simulink model "Control_DC_DC_Test"  (R2018b)
settings: Solver=FixedStepDiscrete  StartTime=0.0  StopTime=1  RelTol=1e-3
undefined symbols (not defined in the file): sigbuilder_block
libraries: powerlib x32, re_lib x1, powerlib_meascontrol x1
settings Model: Creator=jasil  LastModifiedBy=mwkane

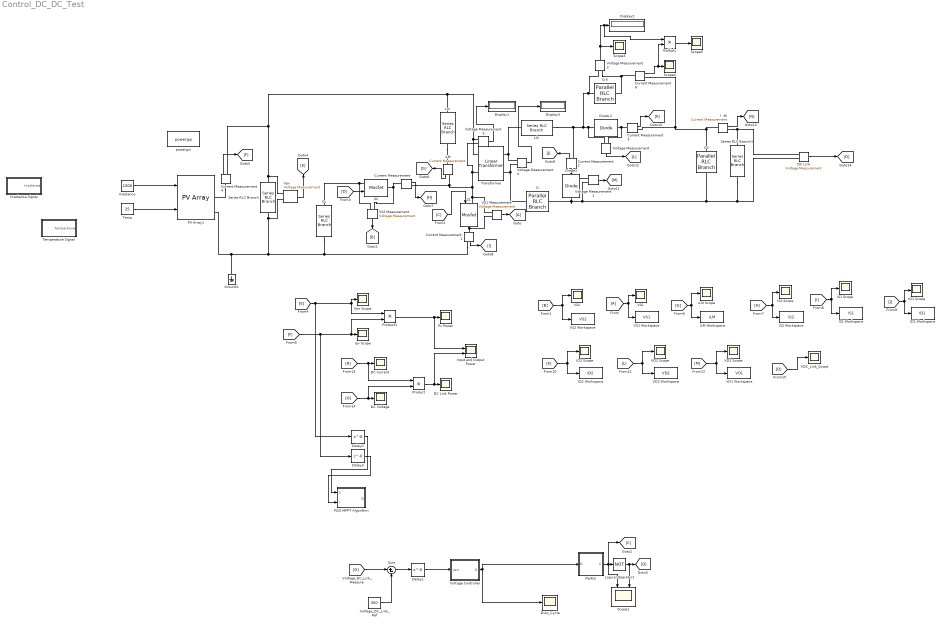
== system Control_DC_DC_Test ==
  " Cd" : powerlib/Elements/Parallel RLC Branch  LConnTagsString=a  RConnTagsString=__new0  BranchType=C  Resistance=1  Inductance=1e-3  SetiL0=off  InitialCurrent=0  Capacitance=1e-5  Setx0=off  InitialVoltage=0  Measurements=None
      settings: SourceProductName=Simscape Electrical
  Cc : powerlib/Elements/Series RLC Branch  LConnTagsString=__new0  RConnTagsString=__new0  BranchType=RC  Resistance=0.001  Inductance=1e-3  SetiL0=off  InitialCurrent=0  Capacitance=2.2e-6  Setx0=off  InitialVoltage=0  Measurements=None
      settings: SourceProductName=Simscape Electrical
  Cr : powerlib/Elements/Parallel RLC Branch  LConnTagsString=a  RConnTagsString=__new0  BranchType=C  Resistance=1  Inductance=1e-3  SetiL0=off  InitialCurrent=0  Capacitance=2.4e-6  Setx0=off  InitialVoltage=0  Measurements=None
      settings: SourceProductName=Simscape Electrical
  Cr3 : powerlib/Elements/Parallel RLC Branch  LConnTagsString=a  RConnTagsString=__new0  BranchType=R  Resistance=1e3  Inductance=2.6e-6  SetiL0=off  InitialCurrent=0  Capacitance=2.4e-6  Setx0=off  InitialVoltage=0  Measurements=None
      settings: SourceProductName=Simscape Electrical
  Current Measurement{,1..4,6} (6 alike) : powerlib/Measurements/Current Measurement  PhasorSimulation=off  OutputType=Complex  PSBequivalent=0
      settings: SourceProductName=Simscape Electrical
  DC Current : Scope
  DC Link : powerlib/Measurements/Voltage Measurement  PhasorSimulation=off  OutputType=Complex  PSBequivalent=0
      settings: SourceProductName=Simscape Electrical
  DC Link Power : Scope
  DC Voltage : Scope
  Delay1 : Delay  DelayLength=0  SampleTime=0.0001
  Delay2 : Delay  DelayLength=0  SampleTime=0.001
  Delay3 : Delay  DelayLength=0  SampleTime=0.001
  Diode 2 : powerlib/Power Electronics/Diode  Ron=1  Lon=0  Vf=0.8  IC=0  UseSnubber=0  Rs=inf  Cs=0  Measurements=off
      settings: SourceProductName=Simscape Electrical
  Diode1 : powerlib/Power Electronics/Diode  Ron=0.01  Lon=0  Vf=0.8  IC=0  UseSnubber=0  Rs=inf  Cs=0  Measurements=off
      settings: SourceProductName=Simscape Electrical
  Display1 : Display
  Display2 : Display
  Display3 : Display
  Duty_Cycle : Scope
  Ground1 : powerlib/Elements/Ground  LConnTagsString=a
      settings: SourceProductName=Simscape Electrical
  I  dc : powerlib/Measurements/Current Measurement  PhasorSimulation=off  OutputType=Complex  PSBequivalent=0
      settings: SourceProductName=Simscape Electrical
  ID1 Scope : Scope
  ID1 Workspace : ToWorkspace  VariableName=ID1  SaveFormat=Timeseries  SampleTime=-1
  ID2 Scope : Scope
  ID2 Workspace : ToWorkspace  VariableName=ID2  SaveFormat=Timeseries  SampleTime=-1
  ILM Workspace : ToWorkspace  VariableName=ILM  SaveFormat=Timeseries  SampleTime=-1
  IS1 Scope : Scope
  IS1 Workspace : ToWorkspace  VariableName=IS1  SaveFormat=Timeseries  SampleTime=-1
  IS2 Scope : Scope
  IS2 Workspace : ToWorkspace  VariableName=IS2  SaveFormat=Timeseries  SampleTime=-1
  Input and Output Power : Scope  NumInputPorts=2
  Ipv Scope : Scope
  Irradiance : Constant  Value=1000
  "Irradiance Signal " : Subsystem  Tag=STV Subsys  LoadFcn=sigbuilder_block('load');  StartFcn=sigbuilder_block('start');  StopFcn=sigbuilder_block('stop');  ClipboardFcn=sigbuilder_block('clipboard');  mask(Sigbuilder block){tuvar=[0:10]}
      mask help: Simulink:masks:SigbuilderBlock_MD
      mask init:
      | if ~strcmp(get_param(bdroot(gcbh),'SimulationStatus'),'stopped') tuvar = sigbuilder_block('maskInit'); end
      settings: CopyFcn=sigbuilder_block('copy');  DeleteFcn=sigbuilder_block('delete');  ModelCloseFcn=sigbuilder_block('modelClose');  PreSaveFcn=sigbuilder_block('preSave');  PauseFcn=sigbuilder_block('pause');  ContinueFcn=sigbuilder_block('continue');  NameChangeFcn=sigbuilder_block('namechange');  OpenFcn=sigbuilder_block('open',[6 30 1012.5 447.75 ]);  CloseFcn=sigbuilder_block('close');
      mask Display: plot(0, 0, 100, 100,[2, 2, 32, 32, 2], [68, 8, 8, 68, 68],[32, 2], [38, 38], [32, 19, 2],[53, 60, 44], [32, 17, 17, 2],[16, 16, 31, 31]);txt = getActiveGroup(gcbh);text(2, 100, txt,'verticalAlignment', 'top');
  Llk : powerlib/Elements/Series RLC Branch  LConnTagsString=__new0  RConnTagsString=__new0  BranchType=RL  Resistance=0.001  Inductance=2.6e-6  SetiL0=off  InitialCurrent=0  Capacitance=1e-6  Setx0=off  InitialVoltage=0  Measurements=None
      settings: SourceProductName=Simscape Electrical
  Lm : powerlib/Elements/Series RLC Branch  LConnTagsString=__new0  RConnTagsString=__new0  BranchType=RL  Resistance=0.001  Inductance=20e-6  SetiL0=off  InitialCurrent=0  Capacitance=1e-6  Setx0=off  InitialVoltage=0  Measurements=None
      settings: SourceProductName=Simscape Electrical
  Logical Operator1 : Logic  Operator=NOT  AllPortsSameDT=off  OutDataTypeStr=boolean
  Multiply : Product
  P&O MPPT Algorithm : MATLAB Function  TreatAsAtomicUnit=on
  PV Array1 : re_lib/Solar/PV Array  Npar=1  Nser=2  PlotType=array @ 25 deg.C & specified irradiances  S_vec="[ 1000  500  100 ]"  Temp_C_vec="[ 45 25  ]"  ModuleName=User-defined  PlotWhenSelected=off  Pm=179.9805  Ncell=36  Voc=24.06  Isc=9.77  Vm=19.67  Im=9.15  beta_Voc_pc=-0.28  alpha_Isc_pc=+0.04  beta_Voc=-0.067368  alpha_Isc=0.003908  IL=9.8911  I0=1.3829e-11  nI=0.95443  Rsh=60.4787  Rs=0.18212  BAL=off  Tc=1e-6  Tfilter=5e-5
      settings: SourceProductName=Simscape Electrical
  PWM2 : Subsystem
  Product : Product
  Product1 : Product
  Pv Power : Scope
  S1 : powerlib/Power Electronics/Mosfet  Ron=5.6e-3  Lon=0  Rd=0.01  Vfd=1.3  IC=0  Rs=1e6  Cs=inf  Measurements=off
      settings: SourceProductName=Simscape Electrical
  S2 : powerlib/Power Electronics/Mosfet  Ron=5.6e-3  Lon=0  Rd=0.01  Vfd=1.3  IC=0  Rs=1e5  Cs=inf  Measurements=off
      settings: SourceProductName=Simscape Electrical
  Scope1 : Scope  NumInputPorts=2
  Scope3 : Scope
  Scope4 : Scope
  Scope5 : Scope
  Series RLC Branch : powerlib/Elements/Series RLC Branch  LConnTagsString=__new0  RConnTagsString=__new0  BranchType=RC  Resistance=0.000001  Inductance=1e-3  SetiL0=off  InitialCurrent=0  Capacitance=1e-3  Setx0=off  InitialVoltage=0  Measurements=Branch voltage
      settings: SourceProductName=Simscape Electrical
  Series RLC Branch1 : powerlib/Elements/Series RLC Branch  LConnTagsString=__new0  RConnTagsString=__new0  BranchType=R  Resistance=695  Inductance=1e-3  SetiL0=off  InitialCurrent=0  Capacitance=1e-6  Setx0=off  InitialVoltage=0  Measurements=None
      settings: SourceProductName=Simscape Electrical
  Sum : Sum  Inputs=|+-
  Temp : Constant  Value=25
  Temperature Signal : Subsystem  Tag=STV Subsys  LoadFcn=sigbuilder_block('load');  StartFcn=sigbuilder_block('start');  StopFcn=sigbuilder_block('stop');  ClipboardFcn=sigbuilder_block('clipboard');  mask(Sigbuilder block){tuvar=[0:10]}
      mask help: Simulink:masks:SigbuilderBlock_MD
      mask init:
      | if ~strcmp(get_param(bdroot(gcbh),'SimulationStatus'),'stopped') tuvar = sigbuilder_block('maskInit'); end
      settings: CopyFcn=sigbuilder_block('copy');  DeleteFcn=sigbuilder_block('delete');  ModelCloseFcn=sigbuilder_block('modelClose');  PreSaveFcn=sigbuilder_block('preSave');  PauseFcn=sigbuilder_block('pause');  ContinueFcn=sigbuilder_block('continue');  NameChangeFcn=sigbuilder_block('namechange');  OpenFcn=sigbuilder_block('open',[6 30 1012.5 447.75 ]);  CloseFcn=sigbuilder_block('close');
      mask Display: plot(0, 0, 100, 100,[2, 2, 32, 32, 2], [68, 8, 8, 68, 68],[32, 2], [38, 38], [32, 19, 2],[53, 60, 44], [32, 17, 17, 2],[16, 16, 31, 31]);txt = getActiveGroup(gcbh);text(2, 100, txt,'verticalAlignment', 'top');
  Transformer : powerlib/Elements/Linear Transformer  UNITS=SI  NominalPower=[ 25 100e3 ]  winding1=[9 0 0]  winding2=[38 0 0]  ThreeWindings=off  winding3=[3.15e+05 3.969e+07 6316.9]  RmLm=[1e6 0]  Measurements=Magnetization current  DataType=on
      settings: SourceProductName=Simscape Electrical
  VD1 Scope : Scope
  VD1 Workspace : ToWorkspace  VariableName=VD1  SaveFormat=Timeseries  SampleTime=-1
  VD2 Scope : Scope
  VD2 Workspace : ToWorkspace  VariableName=VD2  SaveFormat=Timeseries  SampleTime=-1
  VDC_Link_Scope : Scope
  VS1 : Scope
  VS1 Measurement : powerlib/Measurements/Voltage Measurement  PhasorSimulation=off  OutputType=Complex  PSBequivalent=0
      settings: SourceProductName=Simscape Electrical
  VS1 Workspace : ToWorkspace  VariableName=VS1  SaveFormat=Timeseries  SampleTime=-1
  VS2 : Scope
  VS2 Measurement : powerlib/Measurements/Voltage Measurement  PhasorSimulation=off  OutputType=Complex  PSBequivalent=0
      settings: SourceProductName=Simscape Electrical
  VS2 Workspace : ToWorkspace  VariableName=VS2  SaveFormat=Timeseries  SampleTime=-1
  Voltage Controller : MATLAB Function  TreatAsAtomicUnit=on
  Voltage Measurement{,1..4} (5 alike) : powerlib/Measurements/Voltage Measurement  PhasorSimulation=off  OutputType=Complex  PSBequivalent=0
      settings: SourceProductName=Simscape Electrical
  Voltage_DC_Link_Ref : Constant  Value=350
  Vpv : powerlib/Measurements/Voltage Measurement  PhasorSimulation=off  OutputType=Complex  PSBequivalent=0
      settings: SourceProductName=Simscape Electrical
  Vpv Scope : Scope
  iLM : powerlib/Measurements/Current Measurement  PhasorSimulation=off  OutputType=Complex  PSBequivalent=0
      settings: SourceProductName=Simscape Electrical
  iLM Scope : Scope
  powergui : powerlib/powergui  Priority=1  SimulationMode=Discrete  SampleTime=50e-9  frequency=60  Iterations=50  frequencyindice=0  Pbase=100e6  ErrMax=1e-4  UnitsV=kV  UnitsW=MW  buscounter=0  FunctionMessages=off  echomessages=off  EnableUseOfTLC=off  CurrentSourceSwitches=off  DisableSnubberDevices=off  DisableRonSwitches=off  DisableVfSwitches=off  DisplayEquations=off  SolverType=Tustin/Backward Euler (TBE)  Interpol=off  ExternalGateDelay=off  methode=off  Ts=100  x0status=blocks  SPID=on  SwTol=0  HookPort=off  RestoreLinks=warning  ResistiveCurrentMeasurement=off  Frange=[0:2:500]  Ylog=off  Xlog=on  ShowGrid=off  save=off  variable=ZData  structure=0  ZoomFFT=off  StartTime=0.0  cycles=1  DisplayStyle=1  fundamental=60  FreqAxis=off  MaxFrequency=1000  frequencyindicesteady=1  RmsSteady=1  display=off
      settings: SourceProductName=Simscape Electrical
  wires:
  Product1/1 -> Input and Output Power/1, Pv Power/1
  Delay2/1 -> P&O MPPT Algorithm/1(V)
  Delay3/1 -> P&O MPPT Algorithm/2(I)
  PWM2/1(S) -> Scope1/1, [C], Logical Operator1/1
  VS1 Measurement/1 -> [A]
  [A] -> VS1 Workspace/1, VS1/1
  VS2 Measurement/1 -> [B]
  [B] -> VS2 Workspace/1, VS2/1
  Logical Operator1/1 -> Scope1/2, [D]
  [C] -> S1/1
  [D] -> S2/1
  [E] -> Delay2/1, Vpv Scope/1, Product1/1
  [F] -> Product1/2, Ipv Scope/1, Delay3/1
  iLM/1 -> [G]
  [G] -> iLM Scope/1, ILM Workspace/1
  Current Measurement/1 -> [H]
  [H] -> IS2 Workspace/1, IS2 Scope/1
  Current Measurement1/1 -> [I]
  [I] -> IS1 Workspace/1, IS1 Scope/1
  Current Measurement2/1 -> [J]
  [J] -> ID1 Workspace/1, ID1 Scope/1
  Current Measurement3/1 -> [K]
  [K] -> ID2 Workspace/1, ID2 Scope/1
  [L] -> VD2 Workspace/1, VD2 Scope/1
  [M] -> VD1 Workspace/1, VD1 Scope/1
  Voltage Measurement/1 -> [L]
  Voltage Measurement1/1 -> [M]
  DC Link/1 -> [O]
  Vpv/1 -> [E]
  Current Measurement4/1 -> [F]
  I  dc/1 -> [N]
  Product/1 -> Input and Output Power/2, DC Link Power/1
  [O] -> Product/2, DC Voltage/1
  [N] -> Product/1, DC Current/1
  Voltage Measurement2/1 -> Scope3/1, Multiply/1, Display2/1
  Current Measurement6/1 -> Multiply/2, Scope4/1
  Multiply/1 -> Scope5/1
  Voltage Measurement3/1 -> Display1/1
  Voltage Measurement4/1 -> Display3/1
  [O] -> Sum/1
  Voltage_DC_Link_Ref/1 -> Sum/2
  Sum/1 -> Delay1/1
  Delay1/1 -> Voltage Controller/1(Verr)
  Voltage Controller/1(D) -> PWM2/1(D), Duty_Cycle/1
  [O] -> VDC_Link_Scope/1
  Irradiance/1 -> PV Array1/1
  Temp/1 -> PV Array1/2
  connections:
  Current Measurement3/RConn1 -- Current Measurement6/RConn1 -- I  dc/LConn1 -- " Cd"/LConn1
  S1/LConn1 -- VS1 Measurement/LConn1 -- Voltage Measurement3/LConn2 -- Transformer/LConn2 -- Current Measurement/RConn1 -- iLM/RConn1
  Cr/RConn1 -- Voltage Measurement1/LConn2 -- " Cd"/RConn1 -- DC Link/LConn2 -- Series RLC Branch1/RConn1 -- Diode1/LConn1
  Transformer/LConn1 -- Voltage Measurement3/LConn1 -- Lm/LConn1 -- Current Measurement4/RConn1 -- Vpv/LConn1 -- Series RLC Branch/LConn1
  Current Measurement1/RConn1 -- Cc/RConn1 -- Vpv/LConn2 -- Series RLC Branch/RConn1 -- Ground1/LConn1 -- PV Array1/RConn2
  Cr3/LConn1 -- Voltage Measurement2/LConn1 -- Llk/RConn1 -- Current Measurement2/RConn1 -- Voltage Measurement/LConn2 -- Diode 2/LConn1
  I  dc/RConn1 -- Series RLC Branch1/LConn1 -- DC Link/LConn1
  VS2 Measurement/LConn1 -- Cc/LConn1 -- S2/LConn1
  Cr/LConn1 -- Voltage Measurement4/LConn2 -- Transformer/RConn2
  Lm/RConn1 -- iLM/LConn1
  VS2 Measurement/LConn2 -- Current Measurement/LConn1 -- S2/RConn1
  Current Measurement1/LConn1 -- S1/RConn1 -- VS1 Measurement/LConn2
  Current Measurement2/LConn1 -- Diode1/RConn1 -- Voltage Measurement1/LConn1
  Current Measurement3/LConn1 -- Voltage Measurement/LConn1 -- Diode 2/RConn1
  Current Measurement4/LConn1 -- PV Array1/RConn1
  Llk/LConn1 -- Voltage Measurement4/LConn1 -- Transformer/RConn1
  Voltage Measurement2/LConn2 -- Cr3/RConn1 -- Current Measurement6/LConn1

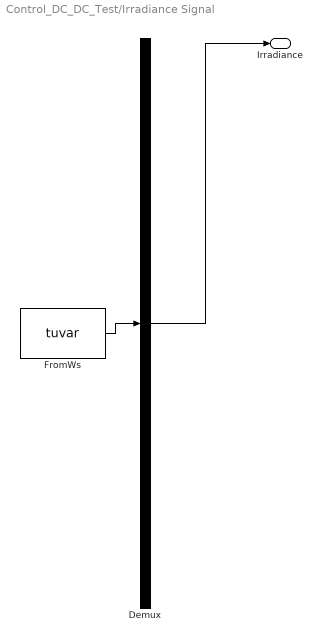
== system Control_DC_DC_Test/Irradiance Signal  ==
  Demux : Demux  Tag=STV Demux  Outputs=1
  FromWs : FromWorkspace  Tag=STV FromWs  VariableName=tuvar  SampleTime=0
      SigBuilderData=|
      | common.afterFinalStr = 'Extrapolate'
      | common.sampleTime = 0
      | dataSet.timeRange = [0 0.3]
      | dataSet.name = 'Group 1'
      | sbobj.Groups.Name = 'Group 1'
      | sbobj.Groups.Signals.Name = 'Irradiance'
      | sbobj.Groups.Signals.XData = [0 0.1 0.1 0.2 0.2 0.3]
      | sbobj.Groups.Signals.YData = [1000 1000 500 500 1000 1000]
      | sbobj.Groups.TimeRange = [0 0.3]
  Irradiance : Outport  Tag=STV Outport
  wires:
  Demux/1 -> Irradiance/1
  FromWs/1 -> Demux/1

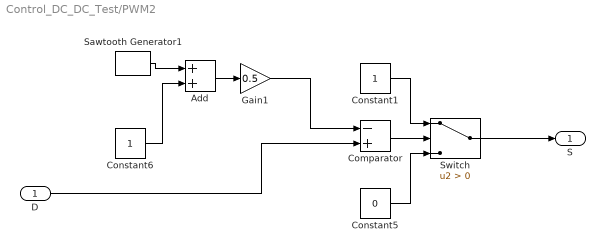
== system Control_DC_DC_Test/PWM2 ==
  D : Inport
  Add : Sum
  Comparator : Sum  Inputs=-+
  Constant1 : Constant
  Constant5 : Constant  Value=0
  Constant6 : Constant
  Gain1 : Gain  Gain=0.5
  Sawtooth Generator1 : powerlib_meascontrol/Pulse & Signal Generators/Sawtooth Generator  Freq=50000  Phase=180  Ts=0
      settings: SourceProductName=Simscape Electrical
  Switch : Switch  Criteria=u2 > Threshold
  S : Outport
  wires:
  Switch/1 -> S/1
  Constant1/1 -> Switch/1
  Comparator/1 -> Switch/2
  Constant6/1 -> Add/2
  Gain1/1 -> Comparator/1
  Constant5/1 -> Switch/3
  Sawtooth Generator1/1 -> Add/1
  Add/1 -> Gain1/1
  D/1 -> Comparator/2

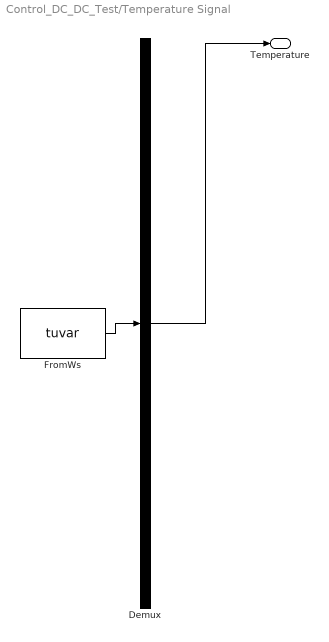
== system Control_DC_DC_Test/Temperature Signal ==
  Demux : Demux  Tag=STV Demux  Outputs=1
  FromWs : FromWorkspace  Tag=STV FromWs  VariableName=tuvar  SampleTime=0
      SigBuilderData=|
      | common.afterFinalStr = 'Extrapolate'
      | common.sampleTime = 0
      | dataSet.timeRange = [0 0.3]
      | dataSet.name = 'Group 1'
      | sbobj.Groups.Name = 'Group 1'
      | sbobj.Groups.Signals.Name = 'Temperature'
      | sbobj.Groups.Signals.XData = [0 0.1 0.1 0.2 0.2 0.3]
      | sbobj.Groups.Signals.YData = [25 25 50 50 25 25]
      | sbobj.Groups.TimeRange = [0 0.3]
  Temperature : Outport  Tag=STV Outport
  wires:
  Demux/1 -> Temperature/1
  FromWs/1 -> Demux/1

== matlab function Control_DC_DC_Test/Voltage Controller ==
  data: Verr input; D output
function D = V_Control(Verr)

persistent d_prev; 

if isempty(d_prev)
    d_prev = 0.75;
end

% Select the change in duty cycle
delta_D = 0.001;

% Increase or decrease duty cycle based on conditions
if(Verr > 0)
    D = d_prev + delta_D;
elseif(Verr < 0)
    D = d_prev - delta_D;
else
    D = d_prev;
end

d_prev = D;

== matlab function Control_DC_DC_Test/P&O MPPT Algorithm ==
  data: V input; D output; I input
function D = PandO(V, I)
persistent p_prev;
persistent v_prev;
persistent d_prev; 


if isempty(d_prev)
    d_prev = 0.69;
    v_prev = 24.06;
    p_prev = 0;
end

% Select the change in duty cycle
delta_D = 0.001;

% Set local variables and calculate pv module power 
Vn = V;
In = I;
Pn = Vn*In;

% Increase or decrease duty cycle based on conditions
if ((Pn - p_prev) ~= 0)
    if ((Pn - p_prev) > 0)
        if ((Vn - v_prev) > 0)
            D = d_prev - delta_D;
        else
            D = d_prev + delta_D;
        end
    else
        if ((Vn - v_prev) > 0)
            D = d_prev + delta_D;
        else
            D = d_prev - delta_D;
        end        
    end
else
    D = d_prev;
end

% Update internal values
d_prev = D;
v_prev = Vn;
p_prev = Pn;
